simulink model "dspsinecomp"  (Simulink 8.3)
settings: Solver=FixedStepDiscrete  StartTime=0.0  StopTime=inf  RelTol=1e-3
libraries: dspsrcs4 x4, dspmisc x1, dspstat3 x1
Description:
  | Comparison of sine wave generation techniques.
settings Model: Creator=The MathWorks Inc.  CovMetricSettings=d  ExtModeTrigMode=oneshot  ExtModeArmWhenConnect=off
settings DataIOCC: LimitDataPoints=off  SaveOutput=off  SaveTime=off
settings OptimizationCC: BlockReduction=off  BooleanDataType=off  ExpressionDepthLimit=2147483647  RollThreshold=2  InitFltsAndDblsToZero=on
settings DebuggingCC: SaveWithParameterizedLinksMsg=none  SignalResolutionControl=TryResolveAllWithWarning  SolverPrmCheckMsg=none  MultiTaskDSMMsg=warning  MultiTaskCondExecSysMsg=none  SingleTaskRateTransMsg=error  IntegerOverflowMsg=none  FcnCallInpInsideContextMsg=UseLocalSettings  StrictBusMsg=None
settings HardwareCC: TargetUnknown=on
settings RTWCC: IncludeERTFirstTime=on
settings GRTTargetCC: TargetFcnLib=ansi_tfl_tmw.mat

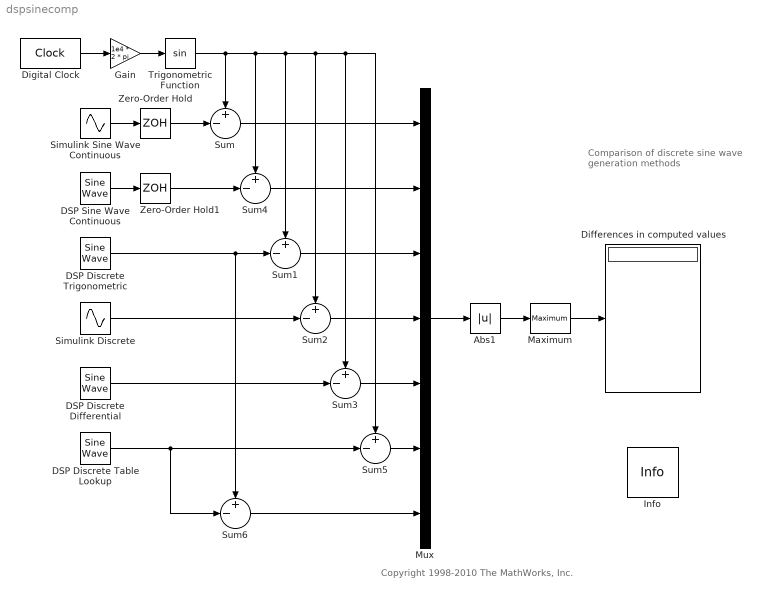
== system dspsinecomp ==
  note: Comparison of discrete
      | sine wave generation methods
  note: Copyright 1998-2010 The MathWorks, Inc.
  Abs1 : Abs  SaturateOnIntegerOverflow=on
  DSP Discrete Differential : dspsrcs4/Sine Wave  Amplitude=1  Frequency=1e4  Phase=0  SampleMode=Discrete  OutComplex=Real  CompMethod=Differential  TableSize=Speed  SampleTime=1e-5  SamplesPerFrame=1  ResetState=Restart at time zero  dataType=double  wordLen=16  udDataType=sfix(16)  fracBitsMode=Best precision  numFracBits=15  OutDataTypeStr=double  LastOutDataTypeStr=double
  DSP Discrete Table Lookup : dspsrcs4/Sine Wave  Amplitude=1  Frequency=1e4  Phase=0  SampleMode=Discrete  OutComplex=Real  CompMethod=Table lookup  TableSize=Speed  SampleTime=1e-5  SamplesPerFrame=1  ResetState=Restart at time zero  dataType=double  wordLen=16  udDataType=sfix(16)  fracBitsMode=Best precision  numFracBits=15  OutDataTypeStr=double  LastOutDataTypeStr=double
  DSP Discrete Trigonometric : dspsrcs4/Sine Wave  Amplitude=1  Frequency=1e4  Phase=0  SampleMode=Discrete  OutComplex=Real  CompMethod=Trigonometric fcn  TableSize=Speed  SampleTime=1e-5  SamplesPerFrame=1  ResetState=Restart at time zero  dataType=double  wordLen=16  udDataType=sfix(16)  fracBitsMode=Best precision  numFracBits=15  OutDataTypeStr=double  LastOutDataTypeStr=double
  DSP Sine Wave Continuous : dspsrcs4/Sine Wave  Amplitude=1  Frequency=1e4  Phase=0  SampleMode=Continuous  OutComplex=Real  CompMethod=Trigonometric fcn  TableSize=Speed  SampleTime=1/1000  SamplesPerFrame=1  ResetState=Restart at time zero  dataType=double  wordLen=16  udDataType=sfix(16)  fracBitsMode=Best precision  numFracBits=15  OutDataTypeStr=double  LastOutDataTypeStr=double
  Differences in computed values : Display
  Digital Clock : DigitalClock  SampleTime=1e-5
  Gain : Gain  Gain=1e4 * 2 * pi  SaturateOnIntegerOverflow=on  OutDataTypeStr=Inherit: Same as input  ParamDataTypeStr=Inherit: Same as input
  Info : dspmisc/Info  SystemSampleTime=-1
  Maximum : dspstat3/Maximum  fcn=Running  reset=None  indexBase=One  operateOver=Each column  Dimension=1  colComp=on  operation=maximum  roiEnable=off  roiType=Rectangles  roiPortion=Entire ROI  roiOutput=Individual statistics for each ROI  roiFlag=off  accumDataTypeStr=Inherit: Same as product output  accumLastDataTypeStr=Inherit: Same as product output  roundingMode=Floor  overflowMode=off
  Mux : Mux  Inputs=7
  Simulink Discrete : Sin  Frequency="1e4  * 2 * pi"  SampleTime=1e-5
  Simulink Sine Wave Continuous : Sin  Frequency=1e4 * 2 * pi  SampleTime=0
  Sum{,1..6} (7 alike) : Sum  Inputs=+-|  SaturateOnIntegerOverflow=on  InputSameDT=on  OutDataTypeStr=Inherit: Same as first input
  Trigonometric Function : Trigonometry
  Zero-Order Hold : ZeroOrderHold  SampleTime=1e-5
  Zero-Order Hold1 : ZeroOrderHold  SampleTime=1e-5
  wires:
  Gain/1 -> Trigonometric Function/1
  Digital Clock/1 -> Gain/1
  Trigonometric Function/1 -> Sum/1, Sum1/1, Sum2/1, Sum3/1, Sum5/1, Sum4/1
  Sum5/1 -> Mux/6
  Sum6/1 -> Mux/7
  DSP Discrete Table Lookup/1 -> Sum5/2, Sum6/2
  Sum3/1 -> Mux/5
  DSP Discrete Differential/1 -> Sum3/2
  Sum2/1 -> Mux/4
  Simulink Discrete/1 -> Sum2/2
  Sum1/1 -> Mux/3
  DSP Discrete Trigonometric/1 -> Sum1/2, Sum6/1
  DSP Sine Wave Continuous/1 -> Zero-Order Hold1/1
  Zero-Order Hold1/1 -> Sum4/2
  Sum4/1 -> Mux/2
  Simulink Sine Wave Continuous/1 -> Zero-Order Hold/1
  Zero-Order Hold/1 -> Sum/2
  Sum/1 -> Mux/1
  Mux/1 -> Abs1/1
  Abs1/1 -> Maximum/1
  Maximum/1 -> Differences in computed values/1
